simulink model "p2_2"  (R2021b)
settings: Solver=VariableStepAuto  StartTime=0.0  StopTime=10000.0  RelTol=1e-3
settings Model: Creator=alimi  LastModifiedBy=alimi

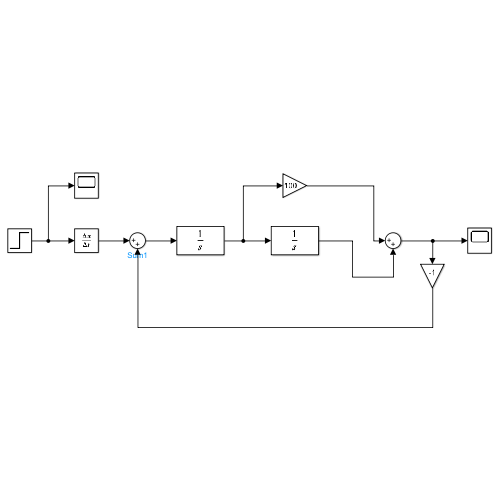
[thumbnail: Simulink's stored preview of the top-level diagram]
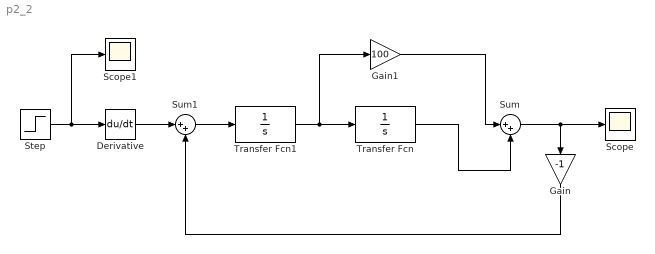
== system p2_2 ==
  Derivative : Derivative
  Gain : Gain  Gain=-1
  Gain1 : Gain  Gain=100
  Scope : Scope
  Scope1 : Scope
  Step : Step  Time=0.001  SampleTime=0
  Sum : Sum  Inputs=|++
  Sum1 : Sum  Inputs=|++
  Transfer Fcn : TransferFcn  Denominator=[1 0]
  Transfer Fcn1 : TransferFcn  Denominator=[1 0]
  wires:
  Sum1/1 -> Transfer Fcn1/1
  Transfer Fcn1/1 -> Gain1/1, Transfer Fcn/1
  Transfer Fcn/1 -> Sum/2
  Sum/1 -> Gain/1, Scope/1
  Gain/1 -> Sum1/2
  Step/1 -> Scope1/1, Derivative/1
  Derivative/1 -> Sum1/1
  Gain1/1 -> Sum/1
